simulink model "HA01"  (R2022b)
settings: Solver=VariableStepAuto  StartTime=0.0  StopTime=50e-3  RelTol=1e-3
values from neighbouring files (symbols this model uses):
  K_I = 1 / J    (= 2380.95238095)    [ParameterHA1.m]
  K_p = 1 / (2 * K_I * T1)    (= 0.06)    [ParameterHA1.m]
  T = 1e-3    (= 0.001)    [ParameterHA1.m]
  T1 = T_EM + T_AH    (= 0.0035)    [ParameterHA1.m]
  T_F = T_n    (= 0.014)    [ParameterHA1.m]
  T_n = 4 * T1    (= 0.014)    [ParameterHA1.m]
settings Model: Creator=hansflottmann  LastModifiedBy=quatj
settings OptimizationCC: ReuseModelBlockBuffer=on
settings RTWCC: GPUComputeCapability=5.0

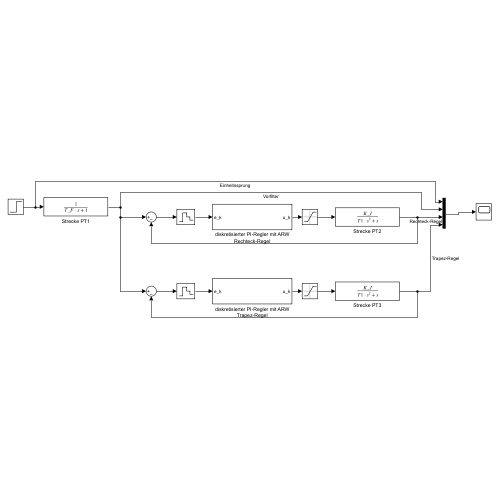
[thumbnail: Simulink's stored preview of the top-level diagram]
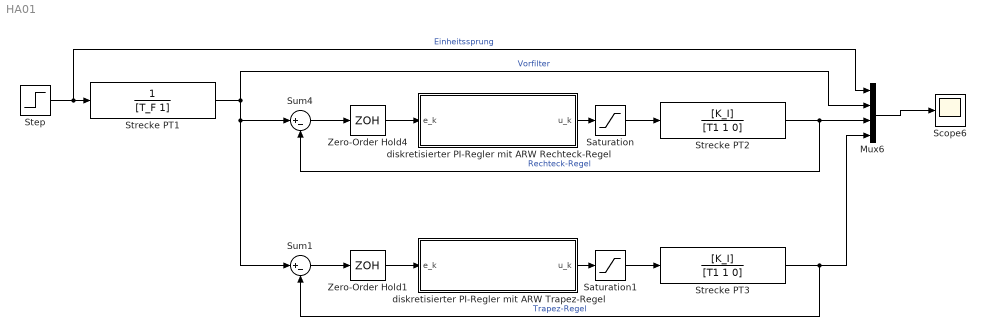
== system HA01 ==
  Mux6 : Mux
  Saturation : Saturate  UpperLimit=4  LowerLimit=-4
  Saturation1 : Saturate  UpperLimit=4  LowerLimit=-4
  Scope6 : Scope
  Step : Step  Time=1e-3  SampleTime=0
  Strecke PT1 : TransferFcn  Denominator=[T_F 1]
  Strecke PT2 : TransferFcn  Numerator=[K_I]  Denominator=[T1 1 0]
  Strecke PT3 : TransferFcn  Numerator=[K_I]  Denominator=[T1 1 0]
  Sum1 : Sum  Inputs=|+-
  Sum4 : Sum  Inputs=|+-
  Zero-Order Hold1 : ZeroOrderHold  SampleTime=T
  Zero-Order Hold4 : ZeroOrderHold  SampleTime=T
  diskretisierter PI-Regler mit ARW Rechteck-Regel : Subsystem
  diskretisierter PI-Regler mit ARW Trapez-Regel : Subsystem
  wires:
  diskretisierter PI-Regler mit ARW Rechteck-Regel/1(u_k) -> Saturation/1
  Strecke PT2/1 -> Mux6/3, Sum4/2  "Rechteck-Regel"
  Mux6/1 -> Scope6/1
  Sum4/1 -> Zero-Order Hold4/1
  Saturation/1 -> Strecke PT2/1
  Zero-Order Hold4/1 -> diskretisierter PI-Regler mit ARW Rechteck-Regel/1(e_k)
  Sum1/1 -> Zero-Order Hold1/1
  diskretisierter PI-Regler mit ARW Trapez-Regel/1(u_k) -> Saturation1/1
  Saturation1/1 -> Strecke PT3/1
  Strecke PT3/1 -> Mux6/4, Sum1/2  "Trapez-Regel"
  Step/1 -> Mux6/1, Strecke PT1/1  "Einheitssprung"
  Zero-Order Hold1/1 -> diskretisierter PI-Regler mit ARW Trapez-Regel/1(e_k)
  Strecke PT1/1 -> Mux6/2, Sum1/1, Sum4/1  "Vorfilter"

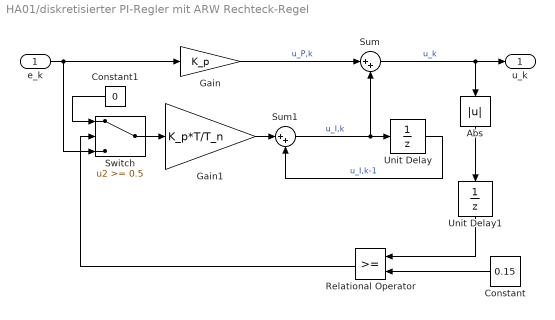
== system HA01/diskretisierter PI-Regler mit ARW Rechteck-Regel ==
  e_k : Inport
  Abs : Abs  SaturateOnIntegerOverflow=off
  Constant : Constant  Value=0.15
  Constant1 : Constant  Value=0
  Gain : Gain  Gain=K_p
  Gain1 : Gain  Gain=K_p*T/T_n
  Relational Operator : RelationalOperator  OutDataTypeStr=boolean  SampleTime=T  InputSameDT=off
  Sum : Sum  Inputs=|++
  Sum1 : Sum  Inputs=|++
  Switch : Switch  Threshold=0.5  SampleTime=T  SaturateOnIntegerOverflow=off  InputSameDT=off
  Unit Delay : UnitDelay  SampleTime=T  HasFrameUpgradeWarning=on
  Unit Delay1 : UnitDelay  SampleTime=T  HasFrameUpgradeWarning=on
  u_k : Outport
  wires:
  Unit Delay/1 -> Sum1/2  "u_I,k-1"
  Sum/1 -> u_k/1, Abs/1  "u_k"
  Gain1/1 -> Sum1/1
  Gain/1 -> Sum/1  "u_P,k"
  Sum1/1 -> Sum/2, Unit Delay/1  "u_I,k"
  e_k/1 -> Switch/3, Gain/1
  Constant/1 -> Relational Operator/2
  Switch/1 -> Gain1/1
  Relational Operator/1 -> Switch/2
  Constant1/1 -> Switch/1
  Unit Delay1/1 -> Relational Operator/1
  Abs/1 -> Unit Delay1/1

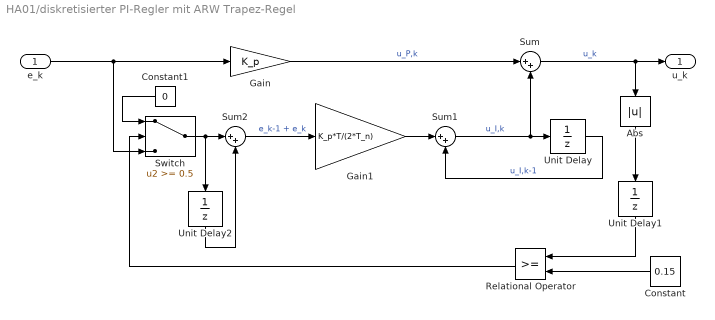
== system HA01/diskretisierter PI-Regler mit ARW Trapez-Regel ==
  e_k : Inport
  Abs : Abs  SaturateOnIntegerOverflow=off
  Constant : Constant  Value=0.15
  Constant1 : Constant  Value=0
  Gain : Gain  Gain=K_p
  Gain1 : Gain  Gain=K_p*T/(2*T_n)
  Relational Operator : RelationalOperator  OutDataTypeStr=boolean  SampleTime=T  InputSameDT=off
  Sum : Sum  Inputs=|++
  Sum1 : Sum  Inputs=|++
  Sum2 : Sum  Inputs=|++
  Switch : Switch  Threshold=0.5  SampleTime=T  SaturateOnIntegerOverflow=off  InputSameDT=off
  Unit Delay : UnitDelay  SampleTime=T  HasFrameUpgradeWarning=on
  Unit Delay1 : UnitDelay  SampleTime=T  HasFrameUpgradeWarning=on
  Unit Delay2 : UnitDelay  SampleTime=T  HasFrameUpgradeWarning=on
  u_k : Outport
  wires:
  Unit Delay/1 -> Sum1/2  "u_I,k-1"
  Sum/1 -> u_k/1, Abs/1  "u_k"
  Gain1/1 -> Sum1/1
  Gain/1 -> Sum/1  "u_P,k"
  Sum1/1 -> Sum/2, Unit Delay/1  "u_I,k"
  e_k/1 -> Switch/3, Gain/1
  Constant/1 -> Relational Operator/2
  Relational Operator/1 -> Switch/2
  Constant1/1 -> Switch/1
  Unit Delay1/1 -> Relational Operator/1
  Abs/1 -> Unit Delay1/1
  Switch/1 -> Unit Delay2/1, Sum2/1
  Sum2/1 -> Gain1/1  "e_k-1 + e_k"
  Unit Delay2/1 -> Sum2/2
